simulink model "Exercise3b"  (Simulink 6.1)
settings: Solver=ode45  StartTime=0.0  StopTime=10.0  RelTol=1e-3
settings Model: LastModifiedBy=Inderjot
settings DebuggingCC: SolverPrmCheckMsg=warning

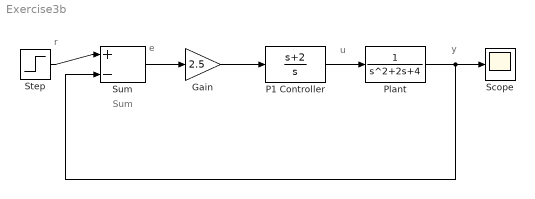
== system Exercise3b ==
  note: Sum
  note: r
  note: e
  note: u
  note: y
  Gain : Gain  Gain=2.5
  P1 Controller : TransferFcn  Numerator=[1 2]  Denominator=[1 0]
  Plant : TransferFcn  Denominator=[1 2 4]
  Scope : Scope
  Step : Step  SampleTime=0
  Sum : Sum  Inputs=|+-
  wires:
  Step/1 -> Sum/1
  Sum/1 -> Gain/1
  Gain/1 -> P1 Controller/1
  P1 Controller/1 -> Plant/1
  Plant/1 -> Scope/1, Sum/2
